simulink model "color_based_seg"  (R2020b)
settings: Solver=FixedStepDiscrete  StartTime=0.0  StopTime=Inf  RelTol=1e-3
libraries: androiduilib x5, androidaudiovideolib x2, visionstatistics x1, visiontextngfix x1
settings Model: Creator=NAYANESH  LastModifiedBy=NAYANESH
settings DataIOCC: ReturnWorkspaceOutputs=off
settings OptimizationCC: EnhancedBackFolding=on  PassReuseOutputArgsThreshold=0  MaxStackSize=64  OptimizeBlockOrder=speed  DifferentSizesBufferReuse=on  OptimizationCustomize=off
settings DebuggingCC: ParameterTunabilityLossMsg=error  ArithmeticOperatorsInVariantConditions=warning
settings HardwareCC: ProdBitPerPointer=32  ProdBitPerSizeT=32  ProdBitPerPtrDiffT=32  ProdLargestAtomicInteger=Long  ProdLargestAtomicFloat=Double  ProdWordSize=32  ProdHWDeviceType=ARM Compatible->ARM Cortex  UseEmbeddedCoderFeatures=off
settings SFSimCC: MATLABDynamicMemAlloc=off  CustomCodeUndefinedFunction=UseInterfaceOnly
settings RTWCC: Description=Embedded Coder  SystemTargetFile=ert.tlc  HardwareBoard=Android Device  TLCOptions="-aInlineSetEventsForThisBaseRateFcn=TLC_FALSE -aSuppressMultiTaskScheduler=TLC_FALSE  -aRateBasedStepFcn=0"  TemplateMakefile=ert_default_tmf  GenerateReport=on  RTWVerbose=off  Toolchain=Android SDK/NDK Tools  LaunchReport=on
settings CodeAppCC: ForceParamTrailComments=on  OperatorAnnotations=on
settings ERTTargetCC: ERTCustomFileBanners=off  SupportContinuousTime=on  SupportNonInlinedSFcns=on  RemoveResetFunc=off  ModelStepFunctionPrototypeControlCompliant=off

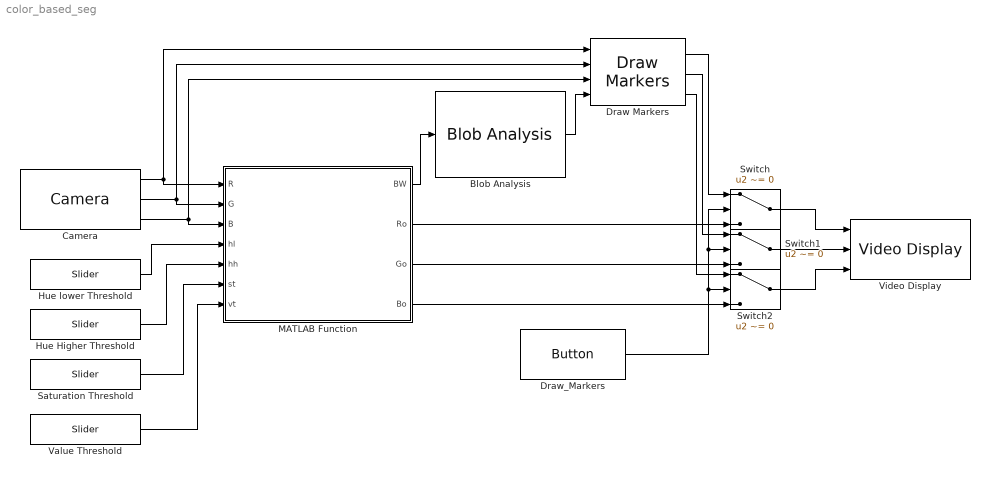
== system color_based_seg ==
  Blob Analysis : visionstatistics/Blob Analysis  Tag=vipblks_row_conv  area=off  centroid=on  bBox=off  majorAxis=off  minorAxis=off  angle=off  eccentricity=off  equivDiameterSq=off  extent=off  perimeter=off  outDT=Specify via Data Types tab  conn=8  isLabel=off  maxBlobs=50  warnIfNumBlobsExceeded=on  isCount=off  useMinArea=off  minArea=0  useMaxArea=off  maxArea=intmax('uint32')  excludeBorderBlob=off  isOutVarDim=off  isFill=on  fillValues=-1  roundingMode=Floor  overflowMode=off  prodOutputMode=Binary point scaling  prodOutputWordLength=32  prodOutputFracLength=16  accumMode=Binary point scaling  accumWordLength=32  accumFracLength=0  outputMode=Binary point scaling  outputWordLength=32  outputFracLength=0  firstCoeffMode=Binary point scaling  firstCoeffWordLength=16  firstCoeffFracLength=14  secondCoeffMode=Binary point scaling  secondCoeffWordLength=32  secondCoeffFracLength=16
  Camera : androidaudiovideolib/Camera  CameraLocation=Back  CameraResolutions=Back - 640x480  Width=640  Height=480  SampleTime=0.001  BlockPlatform=Android
      settings: SourceProductBaseCode=ANDROID
  Draw Markers : visiontextngfix/Draw Markers  shape=Circle  size=3  fill=off  fillClrSource=Specify via dialog  display=User-specified value  intensity=200  color=[255 0 0]  opacity=0.6  viewport=Entire image  antialiasing=off  inType=Obsolete  imagePorts=Separate color signals  roundingMode=Floor  overflowMode=off  memoryMode=Specify word length  memoryWordLength=16  memoryFracLength=15  prodOutputMode=Binary point scaling  prodOutputWordLength=32  prodOutputFracLength=14
      settings: SourceProductBaseCode=VP
  Draw_Markers : androiduilib/Button  ButtonState=Not pressed  ButtonId=color_based_seg/Draw_Markers  State=off  SampleTime=0.001  BlockPlatform=Android
      settings: SourceProductBaseCode=ANDROID
  Hue Higher Threshold : androiduilib/Slider  Min=0  Value=360  Max=360  Resolution=1  SliderId=color_based_seg/Hue_Higher_Threshold  SampleTime=0.001  BlockPlatform=Android
      settings: SourceProductBaseCode=ANDROID
  Hue lower Threshold : androiduilib/Slider  Min=0  Value=0  Max=360  Resolution=1  SliderId=color_based_seg/Hue_lower_Threshold  SampleTime=0.001  BlockPlatform=Android
      settings: SourceProductBaseCode=ANDROID
  MATLAB Function : MATLAB Function  TreatAsAtomicUnit=on
  Saturation Threshold : androiduilib/Slider  Min=0  Value=0  Max=1  Resolution=0.05  SliderId=color_based_seg/Saturation_Threshold  SampleTime=0.001  BlockPlatform=Android
      settings: SourceProductBaseCode=ANDROID
  Switch : Switch  Criteria=u2 ~= 0
  Switch1 : Switch  Criteria=u2 ~= 0
  Switch2 : Switch  Criteria=u2 ~= 0
  Value Threshold : androiduilib/Slider  Min=0  Value=0  Max=1  Resolution=0.05  SliderId=color_based_seg/Value_Threshold  SampleTime=0.001  BlockPlatform=Android
      settings: SourceProductBaseCode=ANDROID
  Video Display : androidaudiovideolib/Video Display  BlockPlatform=Android
      settings: SourceProductBaseCode=ANDROID
  wires:
  Camera/1 -> MATLAB Function/1(R), Draw Markers/1
  Camera/2 -> MATLAB Function/2(G), Draw Markers/2
  Camera/3 -> MATLAB Function/3(B), Draw Markers/3
  MATLAB Function/1(BW) -> Blob Analysis/1
  Hue lower Threshold/1 -> MATLAB Function/4(hl)
  Hue Higher Threshold/1 -> MATLAB Function/5(hh)
  Saturation Threshold/1 -> MATLAB Function/6(st)
  Value Threshold/1 -> MATLAB Function/7(vt)
  Blob Analysis/1 -> Draw Markers/4
  MATLAB Function/2(Ro) -> Switch/3
  MATLAB Function/3(Go) -> Switch1/3
  MATLAB Function/4(Bo) -> Switch2/3
  Switch/1 -> Video Display/1
  Switch1/1 -> Video Display/2
  Switch2/1 -> Video Display/3
  Draw Markers/1 -> Switch/1
  Draw Markers/2 -> Switch1/1
  Draw Markers/3 -> Switch2/1
  Draw_Markers/1 -> Switch/2, Switch1/2, Switch2/2

== matlab function color_based_seg/MATLAB Function ==
  data: R input; BW output; G input; B input; hl input; hh input; st input; vt input; Ro output; Go output; Bo output
function [BW,Ro,Go,Bo] = ColorBasedSegmentation(R,G,B,hl,hh,st,vt)

i=cat(3,R,G,B);
I=i;
i=double(i);
i=i./255;
[r,g,b]=imsplit(i);
cmax=max(i,[],[3]);
cmin=min(i,[],[3]);
delta=cmax-cmin;
H=zeros(size(r));

S=H; V=cmax;

for h=1:size(i,1)
    for w=1:size(i,2)
        if delta(h,w)==0
            H(h,w)=0;
        elseif cmax(h,w)==r(h,w)
            H(h,w)=60*mod(((g(h,w)-b(h,w))/delta(h,w)),6);
        elseif cmax(h,w)==g(h,w)
            H(h,w)=60*(((b(h,w)-r(h,w))/delta(h,w))+2);
        elseif cmax(h,w)==b(h,w)
            H(h,w)=60*(((r(h,w)-g(h,w))/delta(h,w))+4);
        end
        
        if cmax(h,w)==0
            S(h,w)=0;
        else 
            S(h,w)=delta(h,w)/cmax(h,w);
        end
    end
end

BW = H>=hl & H<=hh & S>=st & V>=vt;
BW=imopen(BW, strel('disk',4));

[Ro,Go,Bo]=imsplit(I);
Ro(BW==0)=0;
Go(BW==0)=0;
Bo(BW==0)=0;
